simulink model "robot_exp"  (R2016b)
settings: Solver=ode3  StartTime=0.0  StopTime=1000.0  FixedStep=0.3  RelTol=1e-3  EnableMultiTasking=on
libraries: realtime_pacer_lib x2, robotlib x1, instrumentlib x1
settings Model: Creator=esther  LastModifiedBy=esther
settings DataIOCC: SaveFormat=Array
settings OptimizationCC: MaxStackSize=64
settings DebuggingCC: ParameterTunabilityLossMsg=error
settings HardwareCC: ProdBitPerPointer=32  ProdBitPerSizeT=32  ProdBitPerPtrDiffT=32  ProdLargestAtomicFloat=None  ProdIntDivRoundTo=Undefined  ProdEndianess=Unspecified  ProdWordSize=32  ProdHWDeviceType=Generic->Unspecified (assume 32-bit Generic)
settings RTWCC: SystemTargetFile=ert.tlc  HardwareBoard=Robot Operating System (ROS)  TLCOptions="-aInlineSetEventsForThisBaseRateFcn=TLC_FALSE -aSuppressMultiTaskScheduler=TLC_FALSE  -aRateBasedStepFcn=0"  TemplateMakefile=ert_default_tmf  Description=Embedded Coder  GenerateReport=on  RTWVerbose=off  Toolchain=Catkin  IncludeHyperlinkInReport=on  LaunchReport=on  TargetLang=C++  GenerateTraceInfo=on  GenerateTraceReport=on  GenerateTraceReportSl=on  GenerateTraceReportSf=on  GenerateTraceReportEml=on
settings CodeAppCC: ForceParamTrailComments=on  OperatorAnnotations=on  SimulinkDataObjDesc=on  SFDataObjDesc=on  MATLABFcnDesc=on  InsertBlockDesc=on  MATLABSourceComments=on
settings ERTTargetCC: MultiInstanceERTCode=on  CodeInterfacePackaging=C++ class  SupportContinuousTime=on  SupportVariableSizeSignals=on  RootIOFormat=Structure reference

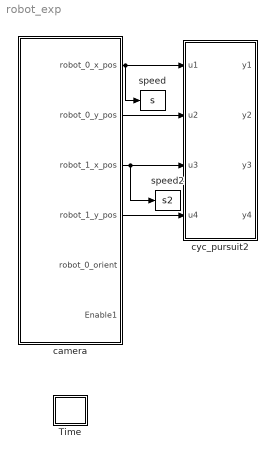
== system robot_exp ==
  Time : Subsystem
  camera : Subsystem
  cyc_pursuit2 : MATLAB Function  TreatAsAtomicUnit=on
  speed : ToWorkspace  VariableName=s  SampleTime=-1
  speed2 : ToWorkspace  VariableName=s2  SampleTime=-1
  wires:
  camera/1(robot_0_x_pos) -> cyc_pursuit2/1(u1), speed/1
  camera/2(robot_0_y_pos) -> cyc_pursuit2/2(u2)
  camera/3(robot_1_x_pos) -> cyc_pursuit2/3(u3), speed2/1
  camera/4(robot_1_y_pos) -> cyc_pursuit2/4(u4)

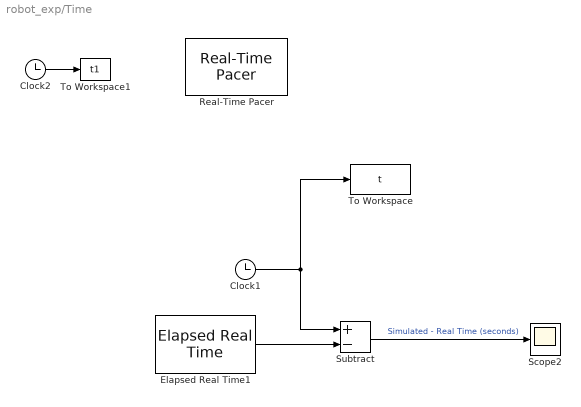
== system robot_exp/Time ==
  Clock1 : Clock
  Clock2 : Clock
  Elapsed Real Time1 : realtime_pacer_lib/Elapsed Real Time
  Real-Time Pacer : realtime_pacer_lib/Real-Time Pacer  simTimePerRealTime=1
  Scope2 : Scope
  Subtract : Sum  Inputs=+-
  To Workspace : ToWorkspace  VariableName=t  SaveFormat=Timeseries  SampleTime=-1
  To Workspace1 : ToWorkspace  VariableName=t1  SampleTime=-1
  wires:
  Elapsed Real Time1/1 -> Subtract/2
  Subtract/1 -> Scope2/1  "Simulated - Real Time (seconds)"
  Clock1/1 -> To Workspace/1, Subtract/1
  Clock2/1 -> To Workspace1/1

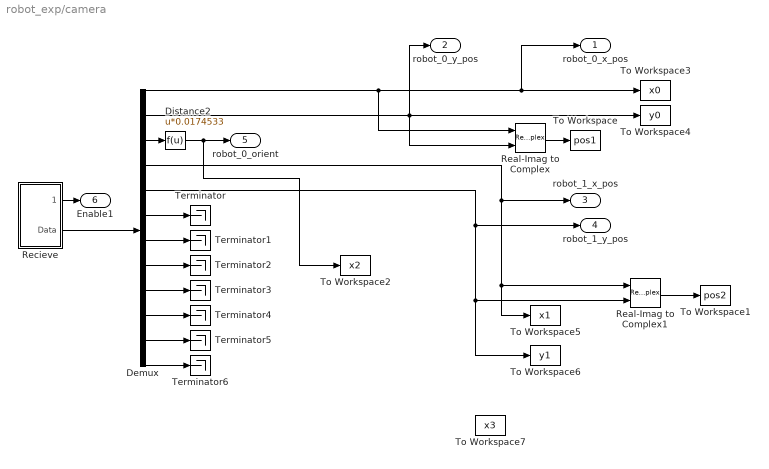
== system robot_exp/camera ==
  Demux : Demux  Outputs=12
  Distance2 : Fcn  Expr=u*0.0174533
  Real-Imag to Complex : RealImagToComplex
  Real-Imag to Complex1 : RealImagToComplex
  Recieve : Subsystem
  Terminator{,1..6} (7 alike) : Terminator
  To Workspace : ToWorkspace  VariableName=pos1  SampleTime=-1
  To Workspace1 : ToWorkspace  VariableName=pos2  SampleTime=-1
  To Workspace2 : ToWorkspace  VariableName=x2  SampleTime=-1
  To Workspace3 : ToWorkspace  VariableName=x0  SampleTime=-1
  To Workspace4 : ToWorkspace  VariableName=y0  SampleTime=-1
  To Workspace5 : ToWorkspace  VariableName=x1  SampleTime=-1
  To Workspace6 : ToWorkspace  VariableName=y1  SampleTime=-1
  To Workspace7 : ToWorkspace  VariableName=x3  SampleTime=-1
  robot_0_x_pos : Outport
  robot_0_y_pos : Outport  Port=2
  robot_1_x_pos : Outport  Port=3
  robot_1_y_pos : Outport  Port=4
  robot_0_orient : Outport  Port=5
  Enable1 : Outport  Port=6
  wires:
  Real-Imag to Complex/1 -> To Workspace/1
  Real-Imag to Complex1/1 -> To Workspace1/1
  Demux/1 -> robot_0_x_pos/1, To Workspace3/1, Real-Imag to Complex/1
  Demux/2 -> Real-Imag to Complex/2, To Workspace4/1, robot_0_y_pos/1
  Demux/6 -> Terminator/1
  Demux/5 -> Real-Imag to Complex1/2, To Workspace6/1, robot_1_y_pos/1
  Demux/4 -> Real-Imag to Complex1/1, To Workspace5/1, robot_1_x_pos/1
  Distance2/1 -> To Workspace2/1, robot_0_orient/1
  Recieve/1(Enable) -> Enable1/1
  Recieve/2(Data) -> Demux/1
  Demux/7 -> Terminator1/1
  Demux/8 -> Terminator2/1
  Demux/9 -> Terminator3/1
  Demux/10 -> Terminator4/1
  Demux/11 -> Terminator5/1
  Demux/12 -> Terminator6/1
  Demux/3 -> Distance2/1

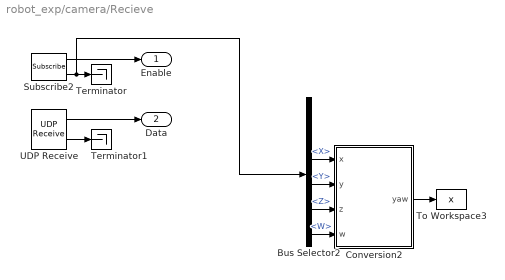
== system robot_exp/camera/Recieve ==
  Bus Selector2 : BusSelector  OutputSignals=Pose.Pose.Position.X,Pose.Pose.Position.Y,Pose.Pose.Orientation.X,Pose.Pose.Orientation.Y,Pose.Pose.Orientation.Z,Pose.Pose.Orientation.W
  Conversion2 : MATLAB Function  TreatAsAtomicUnit=on
  Subscribe2 : robotlib/Subscribe  SourceLibraryInfo=This block requires Robotics System Toolbox  topicSource=Select from ROS network  topic=/robot_0/pose  messageType=nav_msgs/Odometry  sampleTime=-1  messageQueueLength=1
  Terminator : Terminator
  Terminator1 : Terminator
  To Workspace3 : ToWorkspace  VariableName=x  SampleTime=-1
  UDP Receive : instrumentlib/UDP Receive  Host=255.255.255.255  Port=12056  LocalPort=12055  DataSize=12  EnableBlockingMode=off  Timeout=10  SampleTime=-1  DataType=double  ByteOrder=BigEndian
  Enable : Outport
  Data : Outport  Port=2
  wires:
  UDP Receive/1 -> Data/1
  Subscribe2/1 -> Enable/1
  Subscribe2/2 -> Bus Selector2/1, Terminator/1
  UDP Receive/2 -> Terminator1/1
  Bus Selector2/3 -> Conversion2/1(x)  "<X>"
  Bus Selector2/4 -> Conversion2/2(y)  "<Y>"
  Bus Selector2/5 -> Conversion2/3(z)  "<Z>"
  Bus Selector2/6 -> Conversion2/4(w)  "<W>"
  Conversion2/1(yaw) -> To Workspace3/1

== matlab function robot_exp/cyc_pursuit2 ==
  data: u1 input; y1 output; u2 input; u3 input; u4 input; y2 output; y3 output; y4 output
function [y1, y2, y3, y4] = fcn(u1, u2, u3, u4)
%#codegen

y1 = ((1-0.2)*u1+(u3*0.2)-(0.75*0.0));
y2 = ((1-0.2)*u2+(0.2*u4)+(1.2990*0.2));
y3=u1;
y4=u2;




%       y1 = ((1-0.2)*u1+(u3*0.2)+(1.5451*0.2));
%         y2 = ((1-0.2)*u2+(0.2*u4)+(4.7553*0.2));
%         y3 = ((1-0.2)*u3+(u5*0.2)-(4.0451*0.2));
%         y4 = ((1-0.2)*u4+(u6*0.2)+(2.9389*0.2));
%         y5 = ((1-0.2)*u5+(u7*0.2)-(4.0451*0.2));
%         y6 = ((1-0.2)*u6+(u8*0.2)-(2.9389*0.2));
%         y7 = ((1-0.2)*u7+(u9*0.2)+(1.5451*0.2));
%         y8 = ((1-0.2)*u8+(u10*0.2)-(4.7553*0.2));
%         y9 = ((1-0.2)*u9+(u1*0.2)+(5*0.2));
%         y10 = ((1-0.2)*u10+(u2*0.2)+(0*0.2));

== matlab function robot_exp/camera/Recieve/Conversion2 ==
  data: yaw output; x input; y input; z input; w input
function yaw  = quat2eul(x,y,z,w)
%#codegen

% Convert the quaternion to a yaw angle (zyx euler angle)
eul = quat2eul([w,x,y,z]);
yaw = eul(1);

end
